simulink model "PL2_P1_PositionControl"  (R2023b)
settings: Solver=VariableStepAuto  StartTime=0.0  StopTime=10.0  RelTol=1e-3
values from neighbouring files (symbols this model uses):
  refx = 10*rand-5    [PL2_P1_PositionControl_Code.m]
  refy = 10*rand-5    [PL2_P1_PositionControl_Code.m]
undefined symbols (not defined in the file or in its folder): DiscIntNeverNeededParam
libraries: fuzblock x1
settings Model: Creator=lucas  LastModifiedBy=USUARIO
settings DataIOCC: ReturnWorkspaceOutputs=off
settings OptimizationCC: ReuseModelBlockBuffer=off

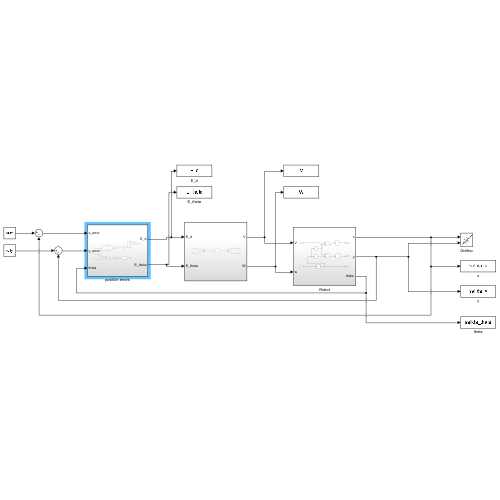
[thumbnail: Simulink's stored preview of the top-level diagram]
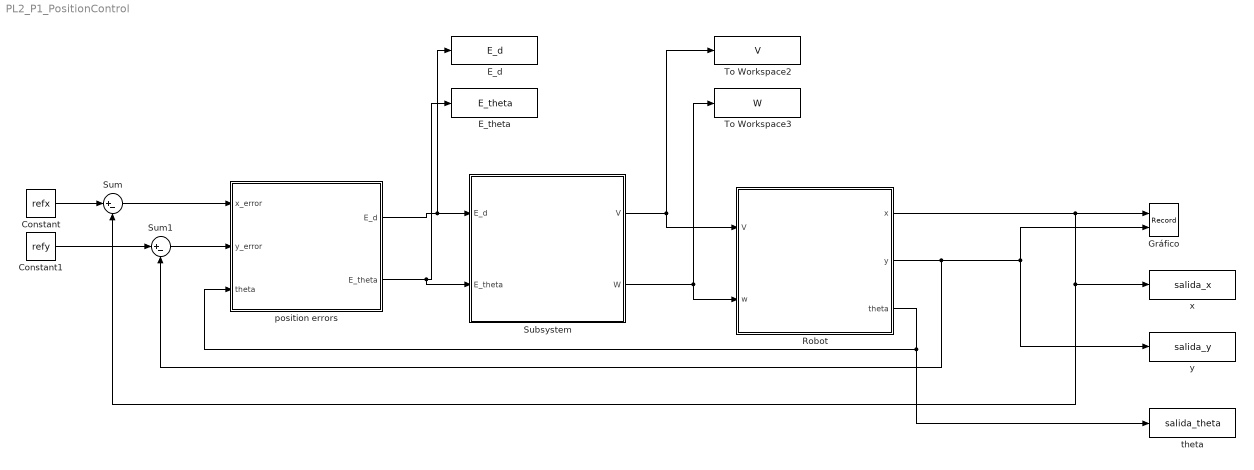
== system PL2_P1_PositionControl ==
  Constant : Constant  Value=refx
  Constant1 : Constant  Value=refy
  E_d : ToWorkspace  VariableName=E_d  SaveFormat=Structure With Time  SampleTime=-1
  E_theta : ToWorkspace  VariableName=E_theta  SaveFormat=Structure With Time  SampleTime=-1
  Gráfico : Record  FileSettingsInternal="{\"entries\":[{\"content\":{\"excelSettings\":{\"content\":{},\"type\":\"Streamout.ExcelSettings\"}},\"type\":\"Streamout.FileSettingStorage\",\"uuid\":\"\"}],\"packageUris\":[\"http:\\/\\/schema.mathworks.com\\/mf0\\/streamout_blocks\\/R2020a\"],\"version\":\"1.0\"}"  Layout=[1 1]  SignalsInternal="{\"entries\":[{\"content\":{\"signals\":[{\"content\":{\"blockPath\":[],\"dimensions\":[1],\"domain\":\"\",\"lineColor\":\"#0072bd\",\"plots\":[1],\"port\":1,\"sid\":[\"\"],\"signalID\":3304,\"signalName\":\"Robot:1\"},\"type\":\"RecordBlkView.Signal\",\"uuid\":\"\"},{\"content\":{\"blockPath\":[],\"dimensions\":[1],\"domain\":\"\",\"lineColor\":\"#d95319\",\"plots\":[1],\"port\":2,\"sid\":[\"\"],\"signalID\":3308,\"signalName\":\"Robot:2\"},\"type\":\"RecordBlkView.Signal\",\"uuid\":\"\"}]},\"type\":\"RecordBlkView.InputSignals\",\"uuid\":\"\"}],\"packageUris\":[\"http:\\/\\/schema.mathworks.com\\/mf0\\/streamout_blocks\\/R2020a\"],\"version\":\"1.0\"}"  VisualizationBindings="{\"xyplotplugin\":{\"info\":[{\"series\":[{\"bindingParametersList\":[{\"parameter\":\"X-Axis\",\"signalID\":3304,\"signalName\":\"Robot:1\"},{\"parameter\":\"Y-Axis\",\"signalID\":3308,\"signalName\":\"Robot:2\"}],\"seriesID\":12571},{\"bindingParametersList\":[{\"parameter\":\"X-Axis\",\"signalID\":3308,\"signalName\":\"Robot:2\"},{\"parameter\":\"Y-Axis\",\"signalID\":3304,\"signalName\":\"Robot:1\"}],\"seriesID\":44487}],\"subplotID\":1}]}}"  CompatibilityTag=XY  st=-1
  Robot : Subsystem
  Subsystem : Subsystem
  Sum : Sum  Inputs=|+-
  Sum1 : Sum  Inputs=|+-
  To Workspace2 : ToWorkspace  VariableName=V  SaveFormat=Structure With Time  SampleTime=-1
  To Workspace3 : ToWorkspace  VariableName=W  SaveFormat=Structure With Time  SampleTime=-1
  position errors : Subsystem
  theta : ToWorkspace  VariableName=salida_theta  SaveFormat=Structure With Time  SampleTime=-1
  x : ToWorkspace  VariableName=salida_x  SaveFormat=Structure With Time  SampleTime=-1
  y : ToWorkspace  VariableName=salida_y  SaveFormat=Structure With Time  SampleTime=-1
  wires:
  Subsystem/2(W) -> To Workspace3/1, Robot/2(w)
  Constant1/1 -> Sum1/1
  Constant/1 -> Sum/1
  Sum/1 -> position errors/1(x_error)
  Sum1/1 -> position errors/2(y_error)
  Subsystem/1(V) -> To Workspace2/1, Robot/1(V)
  Robot/1(x) -> Sum/2, x/1, Gráfico/1
  Robot/2(y) -> Sum1/2, Gráfico/2, y/1
  Robot/3("theta ") -> position errors/3(theta), theta/1
  position errors/1(E_d) -> E_d/1, Subsystem/1(E_d)
  position errors/2(E_theta) -> E_theta/1, Subsystem/2(E_theta)

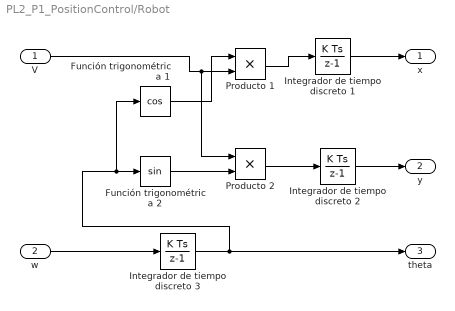
== system PL2_P1_PositionControl/Robot ==
  V : Inport
  w : Inport  Port=2
  Función trigonométrica 1 : Trigonometry  Operator=cos
  Función trigonométrica 2 : Trigonometry
  Integrador de tiempo discreto 1 : DiscreteIntegrator  InitialCondition=-4  SampleTime=0.01  ICPrevOutput=DiscIntNeverNeededParam  ICPrevScaledInput=DiscIntNeverNeededParam
  Integrador de tiempo discreto 2 : DiscreteIntegrator  InitialCondition=-4  SampleTime=0.01  ICPrevOutput=DiscIntNeverNeededParam  ICPrevScaledInput=DiscIntNeverNeededParam
  Integrador de tiempo discreto 3 : DiscreteIntegrator  SampleTime=0.01  ICPrevOutput=DiscIntNeverNeededParam  ICPrevScaledInput=DiscIntNeverNeededParam
  Producto 1 : Product
  Producto 2 : Product
  x : Outport  VectorParamsAs1DForOutWhenUnconnected=off
  y : Outport  Port=2  VectorParamsAs1DForOutWhenUnconnected=off
  "theta " : Outport  Port=3  VectorParamsAs1DForOutWhenUnconnected=off
  wires:
  V/1 -> Producto 2/1, Producto 1/2
  Integrador de tiempo discreto 2/1 -> y/1
  Producto 1/1 -> Integrador de tiempo discreto 1/1
  w/1 -> Integrador de tiempo discreto 3/1
  Función trigonométrica 2/1 -> Producto 2/2
  Producto 2/1 -> Integrador de tiempo discreto 2/1
  Integrador de tiempo discreto 3/1 -> "theta "/1, Función trigonométrica 1/1, Función trigonométrica 2/1
  Integrador de tiempo discreto 1/1 -> x/1
  Función trigonométrica 1/1 -> Producto 1/1

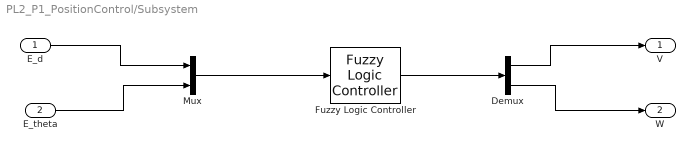
== system PL2_P1_PositionControl/Subsystem ==
  E_d : Inport
  E_theta : Inport  Port=2
  Demux : Demux  Outputs=2
  Fuzzy Logic Controller : fuzblock/Fuzzy Logic  Controller  FIS='ControlBorroso.fis'  OutputSampleNumber=101  DataType=double  FuzzifiedInputs=off  RuleFiringStrengths=off  RuleOutputs=off  AggregatedOutputs=off  SimulateUsing=Interpreted execution  OutOfRangeInputValueMessage=warning  NoRuleFiredMessage=warning  EmptyOutputFuzzySetMessage=warning
  Mux : Mux  Inputs=2
  V : Outport
  W : Outport  Port=2
  wires:
  E_d/1 -> Mux/1
  E_theta/1 -> Mux/2
  Mux/1 -> Fuzzy Logic Controller/1
  Fuzzy Logic Controller/1 -> Demux/1
  Demux/1 -> V/1
  Demux/2 -> W/1

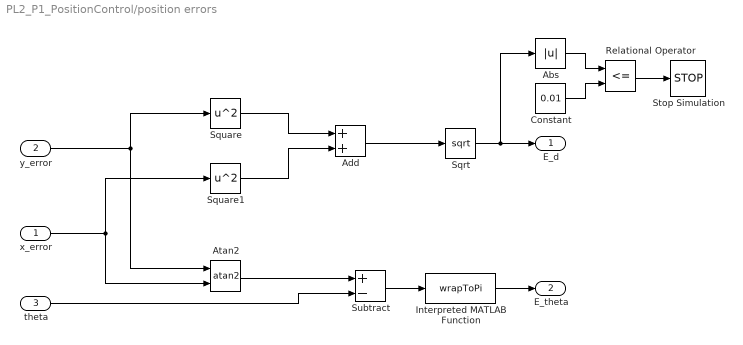
== system PL2_P1_PositionControl/position errors ==
  x_error : Inport
  y_error : Inport  Port=2
  theta : Inport  Port=3
  Abs : Abs  SaturateOnIntegerOverflow=off
  Add : Sum
  Atan2 : Trigonometry  Operator=atan2
  Constant : Constant  Value=0.01
  Interpreted MATLAB Function : MATLABFcn  MATLABFcn=wrapToPi
  Relational Operator : RelationalOperator  Operator=<=  OutDataTypeStr=boolean  RndMeth=Simplest  InputSameDT=off
  Sqrt : Sqrt
  Square : Math  Operator=square  SignedPower=on
  Square1 : Math  Operator=square  SignedPower=on
  Stop Simulation : Stop
  Subtract : Sum  Inputs=+-  OutMin=[-3.14]  OutMax=[3.14]
  E_d : Outport  VectorParamsAs1DForOutWhenUnconnected=off
  E_theta : Outport  Port=2  OutMin=[-pi]  OutMax=[pi]  VectorParamsAs1DForOutWhenUnconnected=off
  wires:
  y_error/1 -> Atan2/1, Square/1
  x_error/1 -> Atan2/2, Square1/1
  Square/1 -> Add/1
  Square1/1 -> Add/2
  Add/1 -> Sqrt/1
  Sqrt/1 -> Abs/1, E_d/1
  Atan2/1 -> Subtract/1
  theta/1 -> Subtract/2
  Abs/1 -> Relational Operator/1
  Constant/1 -> Relational Operator/2
  Relational Operator/1 -> Stop Simulation/1
  Interpreted MATLAB Function/1 -> E_theta/1
  Subtract/1 -> Interpreted MATLAB Function/1
